simulink model "GPS"  (R2021a)
settings: Solver=VariableStepAuto  StartTime=0.0  StopTime=10.0  RelTol=1e-3
undefined symbols (not defined in the file or in its folder): DiscIntNeverNeededParam, Sensor_err
libraries: dspsrcs4 x3
settings Model: Creator=mojta  LastModifiedBy=mojta

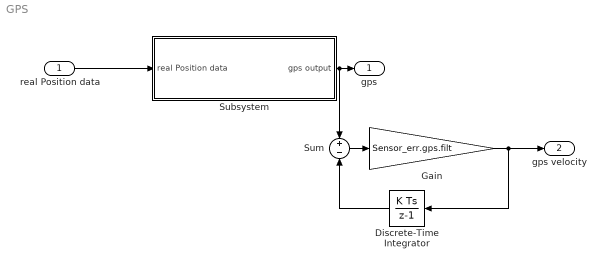
== system GPS ==
  real Position data : Inport  PortDimensions=3
  Discrete-Time Integrator : DiscreteIntegrator  SampleTime=-1  ICPrevOutput=DiscIntNeverNeededParam  ICPrevScaledInput=DiscIntNeverNeededParam
  Gain : Gain  Gain=Sensor_err.gps.filt
  Subsystem : Subsystem
  Sum : Sum  Inputs=+-
  "gps " : Outport
  gps velocity : Outport  Port=2
  wires:
  Subsystem/1(gps output) -> Sum/1, "gps "/1
  real Position data/1 -> Subsystem/1(real Position data)
  Sum/1 -> Gain/1
  Discrete-Time Integrator/1 -> Sum/2
  Gain/1 -> Discrete-Time Integrator/1, gps velocity/1

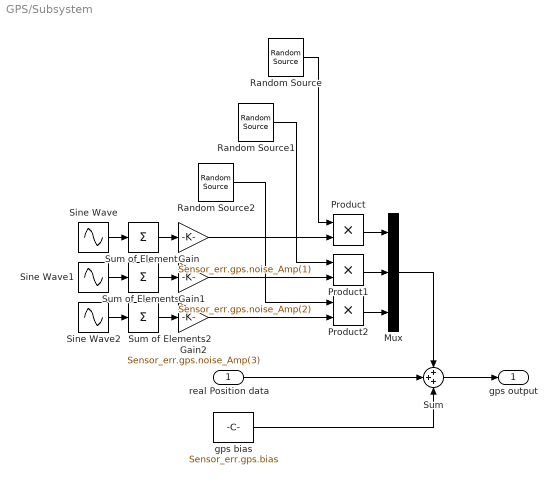
== system GPS/Subsystem ==
  real Position data : Inport
  Gain : Gain  Gain=Sensor_err.gps.noise_Amp(1)
  Gain1 : Gain  Gain=Sensor_err.gps.noise_Amp(2)
  Gain2 : Gain  Gain=Sensor_err.gps.noise_Amp(3)
  Mux : Mux  Inputs=3
  Product : Product
  Product1 : Product
  Product2 : Product
  Random Source : dspsrcs4/Random Source  SrcType=Uniform  NormMethod=Ziggurat  CltLength=12  MinVal=0  MaxVal=1  MeanVal=0  VarVal=1  RepMode=Not repeatable  rawSeed=1  IsInherit=off  SampMode=Discrete  SampTime=1  SampFrame=1  DataType=Double  OutComplex=Real  OutputFrames=off
  Random Source1 : dspsrcs4/Random Source  SrcType=Uniform  NormMethod=Ziggurat  CltLength=12  MinVal=0  MaxVal=1  MeanVal=0  VarVal=1  RepMode=Not repeatable  rawSeed=1  IsInherit=off  SampMode=Discrete  SampTime=1  SampFrame=1  DataType=Double  OutComplex=Real  OutputFrames=off
  Random Source2 : dspsrcs4/Random Source  SrcType=Uniform  NormMethod=Ziggurat  CltLength=12  MinVal=0  MaxVal=1  MeanVal=0  VarVal=1  RepMode=Not repeatable  rawSeed=1  IsInherit=off  SampMode=Discrete  SampTime=1  SampFrame=1  DataType=Double  OutComplex=Real  OutputFrames=off
  Sine Wave : Sin  Frequency=2*pi*Sensor_err.gps.freqs_x  SampleTime=0
  Sine Wave1 : Sin  Frequency=2*pi*Sensor_err.gps.freqs_y  SampleTime=0
  Sine Wave2 : Sin  Frequency=2*pi*Sensor_err.gps.freqs_z  SampleTime=0
  Sum : Sum  Inputs=3
  Sum of Elements : Sum  Inputs=+
  Sum of Elements1 : Sum  Inputs=+
  Sum of Elements2 : Sum  Inputs=+
  gps bias : Constant  Value=Sensor_err.gps.bias
  gps output : Outport
  wires:
  Sum of Elements2/1 -> Gain2/1
  gps bias/1 -> Sum/3
  Sum of Elements1/1 -> Gain1/1
  Sum of Elements/1 -> Gain/1
  Sine Wave/1 -> Sum of Elements/1
  real Position data/1 -> Sum/2
  Sum/1 -> gps output/1
  Sine Wave2/1 -> Sum of Elements2/1
  Sine Wave1/1 -> Sum of Elements1/1
  Gain/1 -> Product/2
  Product1/1 -> Mux/2
  Mux/1 -> Sum/1
  Gain2/1 -> Product2/2
  Random Source2/1 -> Product2/1
  Product2/1 -> Mux/3
  Random Source1/1 -> Product1/1
  Gain1/1 -> Product1/2
  Product/1 -> Mux/1
  Random Source/1 -> Product/1
